simulink model "AM_modulation"  (R2016b)
settings: Solver=VariableStepAuto  StartTime=0.0  StopTime=inf  MaxStep=0.01  RelTol=1e-4  EnableMultiTasking=on
libraries: simulink_extras x4, commsynccomp2 x1
settings Model: Creator=Asus  LastModifiedBy=Asus
settings DataIOCC: LimitDataPoints=on  SaveOutput=off  SaveTime=off
settings OptimizationCC: ExpressionDepthLimit=2147483647  LifeSpan=1
settings DebuggingCC: UnderspecifiedInitializationDetection=Classic  MergeDetectMultiDrivingBlocksExec=none  FcnCallInpInsideContextMsg=warning  AllowSymbolicDim=off  StateNameClashWarn=warning  SFUnexpectedBacktrackingDiag=warning  SFNoUnconditionalDefaultTransitionDiag=warning  SFExecutionAtInitializationDiag=none
settings GRTTargetCC: TargetLangStandard=C89/C90 (ANSI)  GeneratePreprocessorConditionals=Disable all  CombineOutputUpdateFcns=off  GRTInterface=on

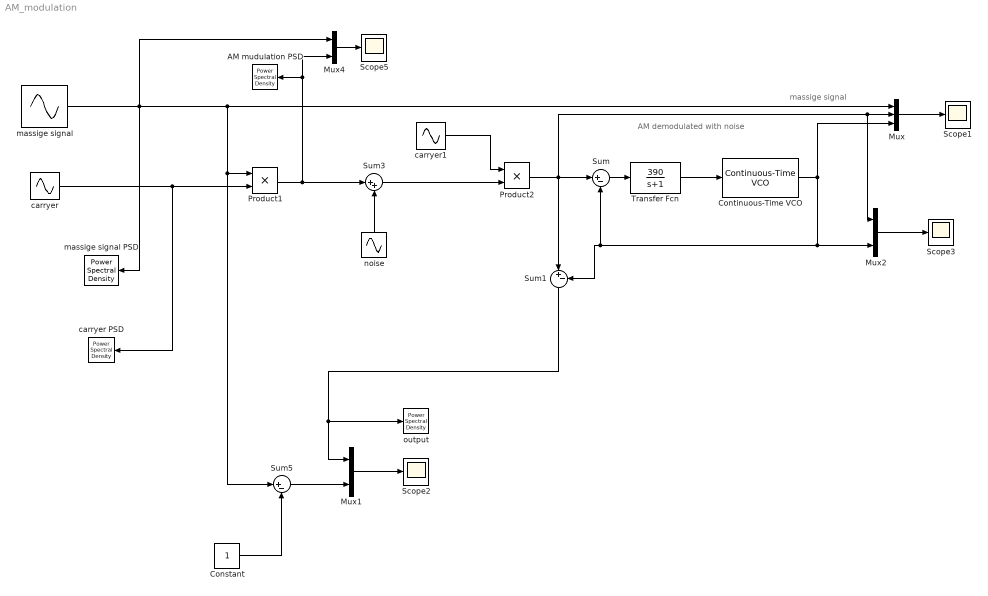
== system AM_modulation ==
  note: AM demodulated with noise
  note: massige signal
  " carryer PSD" : simulink_extras/Additional Sinks/Power Spectral Density  npts=128  fftpts=512  HowOften=64  sampleT=1/45
  AM mudulation PSD : simulink_extras/Additional Sinks/Power Spectral Density  npts=128  fftpts=512  HowOften=64  sampleT=1/45
  Constant : Constant
  Continuous-Time VCO : commsynccomp2/Continuous-Time VCO  Ac=1  Fc=5  Kc=300  Ph=0
  Mux : Mux  Inputs=3
  Mux1 : Mux  Inputs=2
  Mux2 : Mux  Inputs=2
  Mux4 : Mux  Inputs=2
  Product1 : Product
  Product2 : Product
  Scope{1..3,5} (4 alike) : Scope
  Sum : Sum  Inputs=|+-
  Sum1 : Sum  Inputs=|+-
  Sum3 : Sum  Inputs=|++
  Sum5 : Sum  Inputs=|+-
  Transfer Fcn : TransferFcn  Numerator=[390]  Denominator=[1 1]
  carryer : Sin  Frequency=300*2*pi  Phase=pi  SampleTime=0
  carryer1 : Sin  Frequency=300*2*pi  SampleTime=0
  massige signal : Sin  Bias=1  Frequency=5*2*pi  Phase=pi/2  SampleTime=0
  massige signal PSD : simulink_extras/Additional Sinks/Power Spectral Density  npts=128  fftpts=512  HowOften=64  sampleT=1/45
  noise : Sin  Amplitude=0.09  Frequency=85.5*2*pi  SampleTime=0
  output : simulink_extras/Additional Sinks/Power Spectral Density  npts=128  fftpts=512  HowOften=64  sampleT=1/45
  wires:
  Transfer Fcn/1 -> Continuous-Time VCO/1
  Sum/1 -> Transfer Fcn/1
  Mux/1 -> Scope1/1
  Mux1/1 -> Scope2/1
  carryer/1 -> Product1/2, " carryer PSD"/1
  Sum1/1 -> output/1, Mux1/1
  Mux4/1 -> Scope5/1
  Product1/1 -> Mux4/2, AM mudulation PSD/1, Sum3/1
  Constant/1 -> Sum5/2
  Sum3/1 -> Product2/2
  carryer1/1 -> Product2/1
  Sum5/1 -> Mux1/2
  massige signal/1 -> Mux4/1, massige signal PSD/1, Mux/1, Product1/1, Sum5/1
  Mux2/1 -> Scope3/1
  Product2/1 -> Sum/1, Sum1/1, Mux2/1, Mux/2
  Continuous-Time VCO/1 -> Mux/3, Mux2/2, Sum1/2, Sum/2
  noise/1 -> Sum3/2
